simulink model "PID"  (R2024b)
settings: Solver=VariableStepAuto  StartTime=0.0  StopTime=10.0  RelTol=1e-3
settings Model: Creator=MOHAMED  LastModifiedBy=MOHAMED

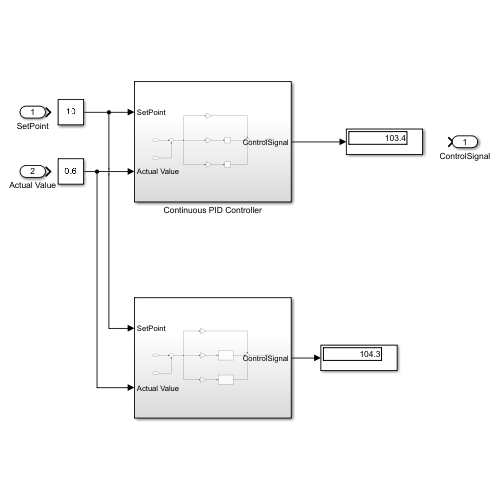
[thumbnail: Simulink's stored preview of the top-level diagram]
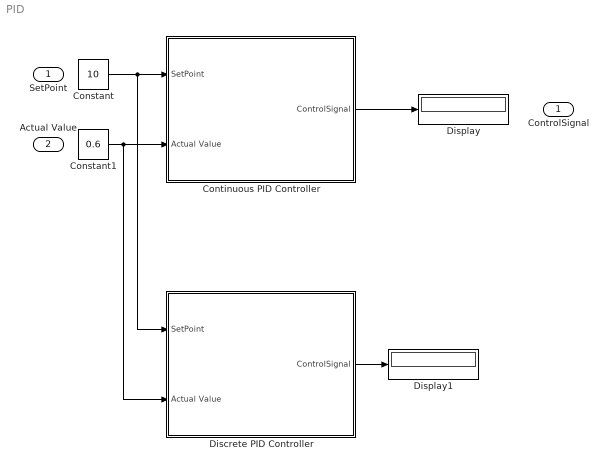
== system PID ==
  SetPoint : Inport
  Actual Value : Inport  Port=2
  Constant : Constant  Value=10
  Constant1 : Constant  Value=0.6
  Continuous PID Controller : Subsystem
  Discrete PID Controller : Subsystem
  Display : Display
  Display1 : Display
  ControlSignal : Outport
  wires:
  Constant/1 -> Discrete PID Controller/1(SetPoint), Continuous PID Controller/1(SetPoint)
  Constant1/1 -> Discrete PID Controller/2(Actual Value), Continuous PID Controller/2(Actual Value)
  Continuous PID Controller/1(ControlSignal) -> Display/1
  Discrete PID Controller/1(ControlSignal) -> Display1/1

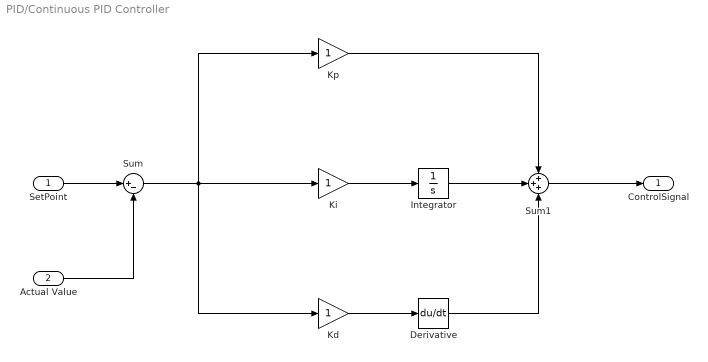
== system PID/Continuous PID Controller ==
  SetPoint : Inport
  Actual Value : Inport  Port=2
  Derivative : Derivative
  Integrator : Integrator
  Kd : Gain
  Ki : Gain
  Kp : Gain
  Sum : Sum  Inputs=|+-
  Sum1 : Sum  Inputs=+++
  ControlSignal : Outport
  wires:
  Ki/1 -> Integrator/1
  Sum1/1 -> ControlSignal/1
  Kp/1 -> Sum1/1
  Actual Value/1 -> Sum/2
  Sum/1 -> Ki/1, Kd/1, Kp/1
  SetPoint/1 -> Sum/1
  Integrator/1 -> Sum1/2
  Derivative/1 -> Sum1/3
  Kd/1 -> Derivative/1

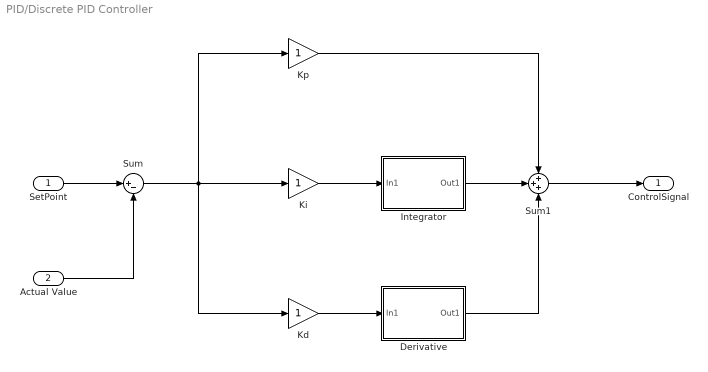
== system PID/Discrete PID Controller ==
  SetPoint : Inport
  Actual Value : Inport  Port=2
  Derivative : Subsystem
  Integrator : Subsystem
  Kd : Gain
  Ki : Gain
  Kp : Gain
  Sum : Sum  Inputs=|+-
  Sum1 : Sum  Inputs=+++
  ControlSignal : Outport
  wires:
  Kd/1 -> Derivative/1(In1)
  Derivative/1(Out1) -> Sum1/3
  Integrator/1(Out1) -> Sum1/2
  SetPoint/1 -> Sum/1
  Sum/1 -> Kp/1, Kd/1, Ki/1
  Actual Value/1 -> Sum/2
  Kp/1 -> Sum1/1
  Sum1/1 -> ControlSignal/1
  Ki/1 -> Integrator/1(In1)

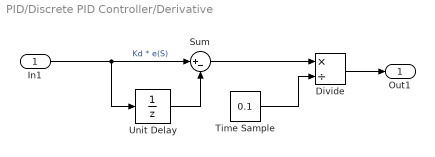
== system PID/Discrete PID Controller/Derivative ==
  In1 : Inport
  Divide : Product  Inputs=*/
  Sum : Sum  Inputs=|+-
  Time Sample : Constant  Value=0.1
  Unit Delay : UnitDelay  SampleTime=0.1  HasFrameUpgradeWarning=on
  Out1 : Outport
  wires:
  In1/1 -> Sum/1, Unit Delay/1  "Kd * e(S)"
  Sum/1 -> Divide/1
  Divide/1 -> Out1/1
  Time Sample/1 -> Divide/2
  Unit Delay/1 -> Sum/2

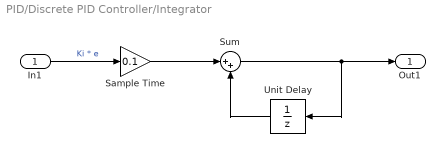
== system PID/Discrete PID Controller/Integrator ==
  In1 : Inport
  Sample Time : Gain  Gain=0.1
  Sum : Sum  Inputs=|++
  Unit Delay : UnitDelay  SampleTime=0.1  HasFrameUpgradeWarning=on
  Out1 : Outport
  wires:
  Sum/1 -> Unit Delay/1, Out1/1
  Unit Delay/1 -> Sum/2
  Sample Time/1 -> Sum/1
  In1/1 -> Sample Time/1  "Ki * e"
